simulink model "electrico_mecanico"  (R2023b)
settings: Solver=VariableStepAuto  StartTime=0.0  StopTime=10.0  RelTol=1e-3
values from neighbouring files (symbols this model uses):
  b = 0.0012    [ELM.m]    (also in ELM_c.m)
  J = 0.001    [ELM.m]    (also in ELM_c.m)
  Ke = 0.01    [ELM.m]    (also in ELM_c.m)
  Kt = 0.01    [ELM.m]    (also in ELM_c.m)
  La = 0.023    [ELM.m]    (also in ELM_c.m)
  Ra = 2    [ELM.m]    (also in ELM_c.m)
settings Model: Creator=mluser

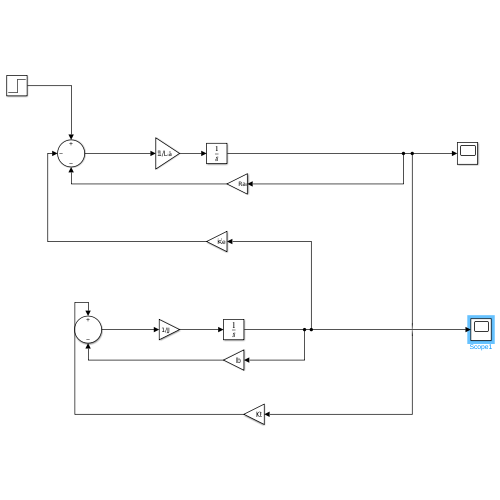
[thumbnail: Simulink's stored preview of the top-level diagram]
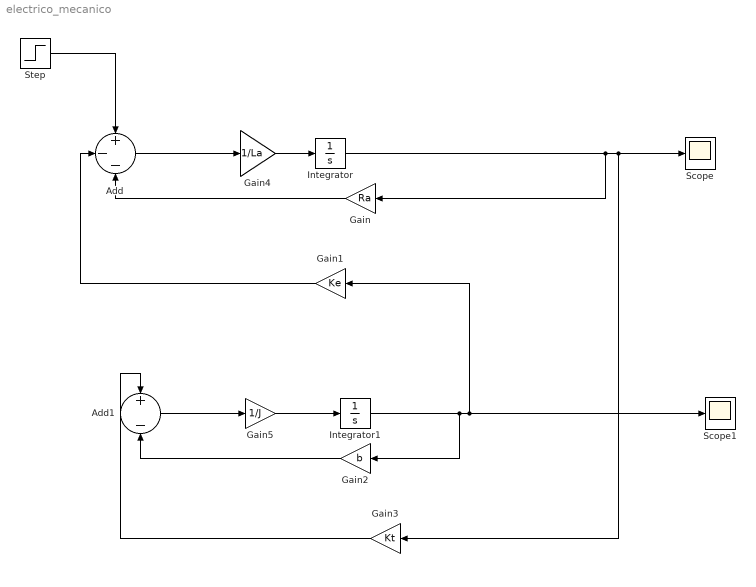
== system electrico_mecanico ==
  Add : Sum  Inputs=+--
  Add1 : Sum  Inputs=+-
  Gain : Gain  Gain=Ra
  Gain1 : Gain  Gain=Ke
  Gain2 : Gain  Gain=b
  Gain3 : Gain  Gain=Kt
  Gain4 : Gain  Gain=1/La
  Gain5 : Gain  Gain=1/J
  Integrator : Integrator
  Integrator1 : Integrator
  Scope : Scope
  Scope1 : Scope
  Step : Step  Time=0  After=5  SampleTime=0
  wires:
  Add/1 -> Gain4/1
  Gain/1 -> Add/3
  Gain1/1 -> Add/2
  Integrator/1 -> Gain/1, Scope/1, Gain3/1
  Add1/1 -> Gain5/1
  Gain2/1 -> Add1/2
  Gain3/1 -> Add1/1
  Gain4/1 -> Integrator/1
  Gain5/1 -> Integrator1/1
  Step/1 -> Add/1
  Integrator1/1 -> Gain2/1, Gain1/1, Scope1/1
